simulink model "lane_pcl_tcpip"  (Simulink 7.1)
settings: Solver=FixedStepDiscrete  SolverMode=SingleTasking  StartTime=0.0  StopTime=inf  RelTol=1e-3
libraries: etargetslib x2, vipsnks x2, instrumentlib x2, dspsrcs4 x1
settings Model: Creator=don  LastModifiedBy=karin  ExtModeAutoUpdateStatusClock=off
settings DataIOCC: SaveOutput=off  SaveTime=off  SignalLoggingName=sigsOut
settings DebuggingCC: CheckExecutionContextPreStartOutputMsg=on  CheckExecutionContextRuntimeOutputMsg=on  SignalResolutionControl=TryResolveAllWithWarning  SolverPrmCheckMsg=none  MultiTaskDSMMsg=warning  MultiTaskCondExecSysMsg=none  ParameterPrecisionLossMsg=none  StrictBusMsg=None
settings HardwareCC: TargetUnknown=on
settings RTWCC: IncludeERTFirstTime=on
settings GRTTargetCC: TargetFcnLib=ansi_tfl_tmw_new.mat

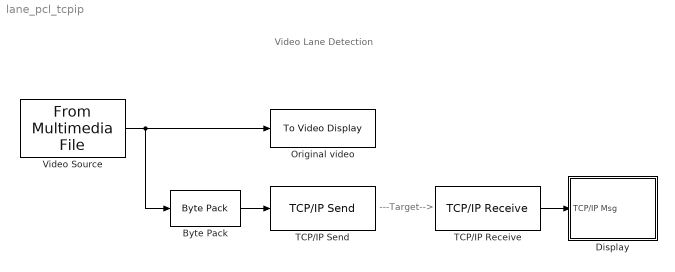
== system lane_pcl_tcpip ==
  note: Video Lane Detection
  note: ---Target-->
  Byte Pack : etargetslib/Byte Pack  datatypes={'uint8'}  byteAlign=1
  Display : Subsystem
  Original video : vipsnks/To Video Display  DialogController=vipDDGCreate  DialogControllerArgs=DataTag1  inputType=Obsolete  imagePorts=One multidimensional signal  OutputDevice=On-screen video monitor  fullScreen=off  videoWindowX=196  videoWindowY=489  saveWindowSize=off  videoWindowWidth=168  videoWindowHeight=147  dataOrg=Column-major
  TCP/IP Receive : instrumentlib/TCP//IP Receive  Priority=10  DialogController=instrumentcreatedialog  DialogControllerArgs=DataTag2  Host=132.66.49.63  Port=49000  DataSize="[1  60480]"  EnableBlockingMode=on  Timeout=6  SampleTime=1/20  DataType=uint8  ByteOrder=BigEndian
  TCP/IP Send : instrumentlib/TCP//IP Send  Priority=5  DialogController=instrumentcreatedialog  DialogControllerArgs=DataTag3  Host=132.66.49.63  Port=49000  EnableBlockingMode=on  Timeout=6  ByteOrder=BigEndian
  Video Source : dspsrcs4/From Multimedia File  Priority=1  DialogController=dspDDGCreate  DialogControllerArgs=DataTag4  inputFilename=viplane_Y.avi  loop=on  numPlays=inf  outputStreams=Video only  videoDataType=uint8  audioDataType=int16  inheritSampleTime=on  userDefinedSampleTime=1/30  noAudioOutput=off  isIntensityVideo=on  colorVideoFormat=Separate color signals  outputEOF=off  dataOrg=Column-major
  wires:
  Video Source/1 -> Original video/1, Byte Pack/1
  Byte Pack/1 -> TCP/IP Send/1
  TCP/IP Receive/1 -> Display/1(TCP/IP Msg)

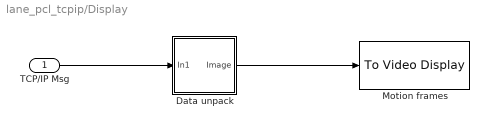
== system lane_pcl_tcpip/Display ==
  TCP/IP Msg : Inport  OutDataType=sfix(16)  OutScaling=2^0
  Data unpack : Subsystem
  Motion frames : vipsnks/To Video Display  DialogController=vipDDGCreate  DialogControllerArgs=DataTag0  inputType=Obsolete  imagePorts=One multidimensional signal  OutputDevice=On-screen video monitor  fullScreen=off  videoWindowX=587  videoWindowY=483  saveWindowSize=off  videoWindowWidth=168  videoWindowHeight=147  dataOrg=Column-major
  wires:
  Data unpack/1(Image) -> Motion frames/1
  TCP/IP Msg/1 -> Data unpack/1(In1)

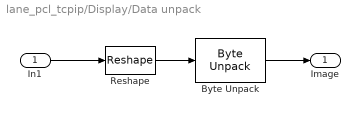
== system lane_pcl_tcpip/Display/Data unpack ==
  In1 : Inport  OutDataType=sfix(16)  OutScaling=2^0
  Byte Unpack : etargetslib/Byte Unpack  dimensions={[168, 360]}  datatypes={'uint8'}  byteAlign=1
  Reshape : Reshape  OutputDimensions=[168,360]
  Image : Outport  OutDataType=sfix(16)  OutScaling=2^0
  wires:
  Reshape/1 -> Byte Unpack/1
  Byte Unpack/1 -> Image/1
  In1/1 -> Reshape/1
